simulink model "pd"  (R2013a)
settings: Solver=ode45  StartTime=0.0  StopTime=10.0  RelTol=1e-6
values from neighbouring files (symbols this model uses):
  k1 = 5    [wiener.m]
  k2 = 0.8    [wiener.m]
  skok = 0    [wiener.m]
settings Model: Creator=L13-4  LastModifiedBy=Dawid Perdek
settings DataIOCC: SignalLoggingSaveFormat=ModelDataLogs
settings DebuggingCC: UnderspecifiedInitializationDetection=Simplified  MultiTaskDSMMsg=warning  MultiTaskCondExecSysMsg=none  StateNameClashWarn=none  StrictBusMsg=ErrorOnBusTreatedAsVector
settings RTWCC: IncludeERTFirstTime=on
settings GRTTargetCC: CodeReplacementLibrary=None  CPPClassGenCompliant=on

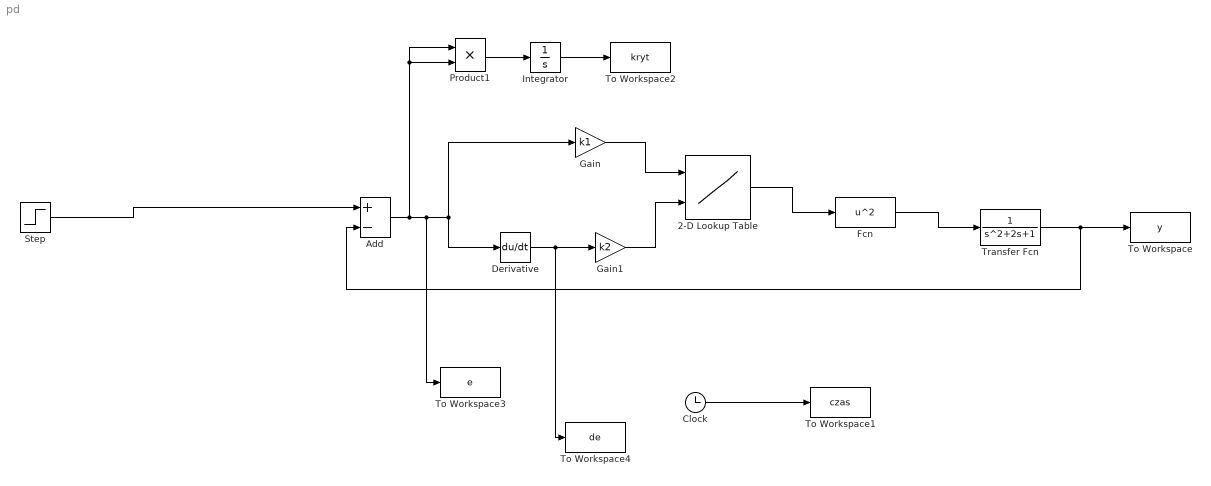
== system pd ==
  2-D Lookup Table : Lookup_n-D  BreakpointsForDimension1=[1:3]  BreakpointsForDimension2=[1:3]  Table=[4 5 6 ; 16 19 20 ; 10 18 23]  RndMeth=Simplest  InputSameDT=on
  Add : Sum  Inputs=+-
  Clock : Clock
  Derivative : Derivative
  Fcn : Fcn  Expr=u^2
  Gain : Gain  Gain=k1
  Gain1 : Gain  Gain=k2
  Integrator : Integrator
  Product1 : Product
  Step : Step  Time=skok  SampleTime=0
  To Workspace : ToWorkspace  VariableName=y  SampleTime=-1
  To Workspace1 : ToWorkspace  VariableName=czas  SampleTime=-1
  To Workspace2 : ToWorkspace  VariableName=kryt  SampleTime=-1
  To Workspace3 : ToWorkspace  VariableName=e  SampleTime=-1
  To Workspace4 : ToWorkspace  VariableName=de  SampleTime=-1
  Transfer Fcn : TransferFcn
  wires:
  Step/1 -> Add/1
  Derivative/1 -> To Workspace4/1, Gain1/1
  Fcn/1 -> Transfer Fcn/1
  Transfer Fcn/1 -> To Workspace/1, Add/2
  Clock/1 -> To Workspace1/1
  Product1/1 -> Integrator/1
  Integrator/1 -> To Workspace2/1
  Add/1 -> Product1/2, Product1/1, To Workspace3/1, Derivative/1, Gain/1
  Gain/1 -> 2-D Lookup Table/1
  Gain1/1 -> 2-D Lookup Table/2
  2-D Lookup Table/1 -> Fcn/1
